simulink model "DDCU_wxt_v02_forA_OpenLoop"  (R2014a)
settings: Solver=FixedStepDiscrete  StartTime=0.0  StopTime=16  FixedStep=0.05  RelTol=1e-3
InitFcn:
  | Veh_Par_wxt
values from neighbouring files (symbols this model uses):
  ag_thr = 0.4*g    (= 3.924)    [Veh_Par_wxt.m]
  B = 2.25    [Veh_Par_wxt.m]
  bra_pre_em = 12    [Veh_Par_wxt.m]
  bra_pre_gz2 = 12/3    (= 4)    [Veh_Par_wxt.m]
  bra_pre_gz34 = 12/3    (= 4)    [Veh_Par_wxt.m]
  bra_pre_yd = 12/2    (= 6)    [Veh_Par_wxt.m]
  brakepre_dem_data = [0 1 2 3 4 5 6 7 8 9 10 11 12]    [Veh_Par_wxt.m]
  brakeTrq_dem_data = [0 218.198 436.396 654.594 872.792 1090.99 1309.188 1527.386 1745.584 1963.782 2181.98 2400.178 2618.376]    [Veh_Par_wxt.m]
  bratrq_max = 4*2618.376    (= 10473.504)    [Veh_Par_wxt.m]
  eff_tran = 0.75    [Veh_Par_wxt.m]
  G = Mass*g    (= 36297)    [Veh_Par_wxt.m]
  kd1 = 1    [Veh_Par_wxt.m]
  kd2 = 1    [Veh_Par_wxt.m]
  kd3 = 1    [Veh_Par_wxt.m]
  ki1 = 1    [Veh_Par_wxt.m]
  ki2 = 1    [Veh_Par_wxt.m]
  ki3 = 1    [Veh_Par_wxt.m]
  kp1 = 1    [Veh_Par_wxt.m]
  kp2 = 1    [Veh_Par_wxt.m]
  kp3 = 1    [Veh_Par_wxt.m]
  L = 3.12    [Veh_Par_wxt.m]
  premax = 12    [Veh_Par_wxt.m]
  Radius = 0.20    (= 0.2)    [Veh_Par_wxt.m]
  s_opt_yi_add = 0.05    [Veh_Par_wxt.m]
  s_opt_zhuan_add = 0.05    [Veh_Par_wxt.m]
  spd_map_mot = [0 100 200 300 360 400 500 600 700 800 900]*tras_ratio    [Veh_Par_wxt.m]
  spdmax = 900*tras_ratio    (= 5580)    [Veh_Par_wxt.m]
  speed_thr_park = 5/3.6/Radius*30/pi    (= 66.3145596216)    [Veh_Par_wxt.m]
  tras_ratio = 6.2    [Veh_Par_wxt.m]
  trq_map_mot = [1200 1200 1200 1200 1200 1080 864 720 617 540 480]/tras_ratio    [Veh_Par_wxt.m]
  trqmax = 80    [Veh_Par_wxt.m]
  v_thr1_b = 5    [Veh_Par_wxt.m]
  v_thr2_b = 20    [Veh_Par_wxt.m]
  v_thr_park = 5    [Veh_Par_wxt.m]
undefined symbols (not defined in the file or in its folder): DiscIntNeverNeededParam, sigbuilder_block
libraries: simulink x169, ec5744lib x9
(part 11 of 13)

== system DDCU_wxt_v02_forA_OpenLoop/MainControl/mode_control/backward/backward/Drive/驱动防滑控制TCS/转向TCS/右转/无滑转 ==
  trq_dem_lf : Inport
  trq_dem_lr : Inport  Port=2
  trq_dem_rf : Inport  Port=3
  trq_dem_rr : Inport  Port=4
  bra_pre_l : Inport  Port=5
  bra_pre_r : Inport  Port=6
  brake_dem : Inport  Port=7
  Action Port : ActionPort  ActionType=case
  1-D Lookup Table : Lookup_n-D  NumberOfTableDimensions=1  BreakpointsForDimension1=brakeTrq_dem_data  Table=brakepre_dem_data  InternalRulePriority=Speed  RndMeth=Simplest  InputSameDT=on
  1-D Lookup Table2 : Lookup_n-D  NumberOfTableDimensions=1  BreakpointsForDimension1=brakeTrq_dem_data  Table=brakepre_dem_data  InternalRulePriority=Speed  RndMeth=Simplest  InputSameDT=on
  Add2 : Sum
  Add3 : Sum
  Constant : Constant  Value=bratrq_max
  Gain1 : Gain  Gain=1/2
  Gain2 : Gain  Gain=1/100
  Gain3 : Gain  Gain=1/2
  Gain4 : Gain  Gain=1/2
  HeartBeat : MATLAB Function  TreatAsAtomicUnit=on
  HeartBeat1 : MATLAB Function  TreatAsAtomicUnit=on
  Memory : Memory  InheritSampleTime=on
  Memory1 : Memory  InheritSampleTime=on
  Mux : Mux  Inputs=8
  Mux1 : Mux  Inputs=8
  Mux2 : Mux  Inputs=7
  Mux3 : Mux  Inputs=7
  Product : Product
  Saturation{,1..3} (4 alike) : Saturate  UpperLimit=trqmax  LowerLimit=-trqmax
  Saturation4 : Saturate  UpperLimit=premax  LowerLimit=0
  Saturation5 : Saturate  UpperLimit=premax  LowerLimit=0
  SpdLim_dem{,1..3} (4 alike) : Constant  Value=spdmax
  SpdSet_dem{,1..3} (4 alike) : Constant
  TrqLim_dem{,1..3} (4 alike) : Constant
  mot_drive : Constant  Value=2
  mot_drive1 : Constant
  mot_drive2 : Constant  Value=2
  mot_drive3 : Constant
  mot_enable{,1..3} (4 alike) : Constant  Value=2
  mot_mode{,1..3} (4 alike) : Constant
  mot_lf : Outport
  mot_lr : Outport  Port=2
  mot_rf : Outport  Port=3
  mot_rr : Outport  Port=4
  bra_pre_l1 : Outport  Port=5
  bra_pre_r1 : Outport  Port=6
  wires:
  Saturation5/1 -> bra_pre_r1/1
  Saturation4/1 -> bra_pre_l1/1
  Saturation3/1 -> Mux3/4
  Saturation2/1 -> Mux2/4
  Saturation1/1 -> Mux1/4
  Saturation/1 -> Mux/4
  brake_dem/1 -> Gain2/1
  Add3/1 -> Saturation5/1
  bra_pre_r/1 -> Add3/2
  1-D Lookup Table2/1 -> Add3/1
  Gain4/1 -> 1-D Lookup Table2/1
  Gain3/1 -> 1-D Lookup Table/1
  Gain2/1 -> Product/2
  Gain1/1 -> Gain3/1, Gain4/1
  Product/1 -> Gain1/1
  Constant/1 -> Product/1
  1-D Lookup Table/1 -> Add2/1
  Add2/1 -> Saturation4/1
  bra_pre_l/1 -> Add2/2
  mot_drive/1 -> Mux/3
  mot_mode/1 -> Mux/2
  trq_dem_lf/1 -> Saturation/1
  mot_enable/1 -> Mux/1
  SpdSet_dem/1 -> Mux/5
  Mux/1 -> mot_lf/1
  TrqLim_dem/1 -> Mux/6
  HeartBeat/1(life) -> Mux/8, Memory/1
  Memory/1 -> HeartBeat/1(life_pre)
  SpdLim_dem/1 -> Mux/7
  mot_drive1/1 -> Mux2/3
  mot_mode2/1 -> Mux2/2
  trq_dem_rf/1 -> Saturation2/1
  mot_enable2/1 -> Mux2/1
  SpdSet_dem1/1 -> Mux2/5
  Mux2/1 -> mot_rf/1
  TrqLim_dem1/1 -> Mux2/6
  SpdLim_dem1/1 -> Mux2/7
  mot_drive2/1 -> Mux1/3
  mot_mode1/1 -> Mux1/2
  trq_dem_lr/1 -> Saturation1/1
  mot_enable1/1 -> Mux1/1
  SpdSet_dem2/1 -> Mux1/5
  Mux1/1 -> mot_lr/1
  TrqLim_dem2/1 -> Mux1/6
  HeartBeat1/1(life) -> Mux1/8, Memory1/1
  Memory1/1 -> HeartBeat1/1(life_pre)
  SpdLim_dem2/1 -> Mux1/7
  mot_drive3/1 -> Mux3/3
  mot_mode3/1 -> Mux3/2
  trq_dem_rr/1 -> Saturation3/1
  mot_enable3/1 -> Mux3/1
  SpdSet_dem3/1 -> Mux3/5
  Mux3/1 -> mot_rr/1
  TrqLim_dem3/1 -> Mux3/6
  SpdLim_dem3/1 -> Mux3/7

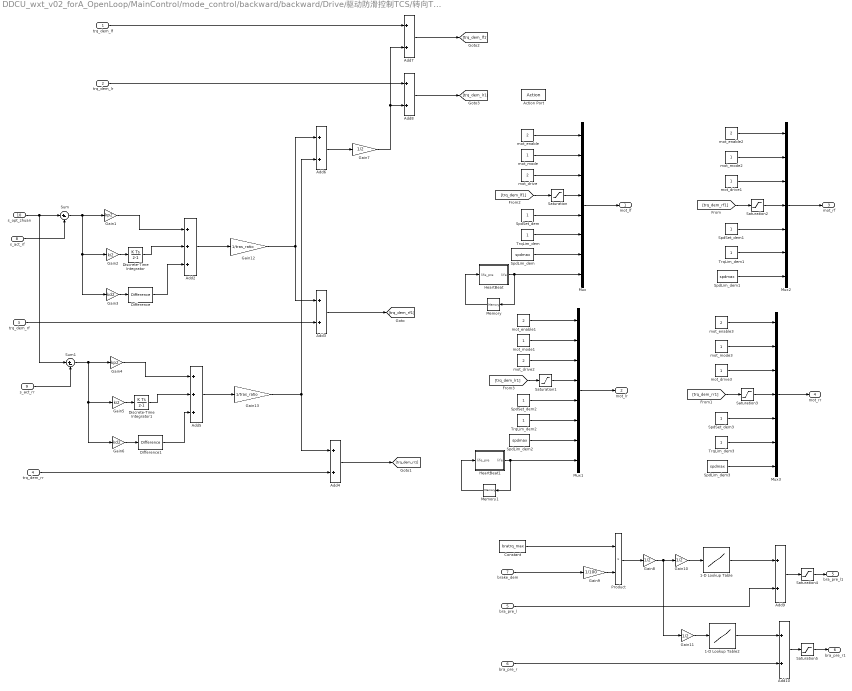
== system DDCU_wxt_v02_forA_OpenLoop/MainControl/mode_control/backward/backward/Drive/驱动防滑控制TCS/转向TCS/左转/前后轮均滑转 ==
  trq_dem_lf : Inport
  trq_dem_lr : Inport  Port=2
  trq_dem_rf : Inport  Port=3
  trq_dem_rr : Inport  Port=4
  bra_pre_l : Inport  Port=5
  bra_pre_r : Inport  Port=6
  brake_dem : Inport  Port=7
  s_act_rf : Inport  Port=8
  s_act_rr : Inport  Port=9
  s_opt_zhuan : Inport  Port=10
  Action Port : ActionPort  ActionType=case
  1-D Lookup Table : Lookup_n-D  NumberOfTableDimensions=1  BreakpointsForDimension1=brakeTrq_dem_data  Table=brakepre_dem_data  InternalRulePriority=Speed  RndMeth=Simplest  InputSameDT=on
  1-D Lookup Table2 : Lookup_n-D  NumberOfTableDimensions=1  BreakpointsForDimension1=brakeTrq_dem_data  Table=brakepre_dem_data  InternalRulePriority=Speed  RndMeth=Simplest  InputSameDT=on
  Add{3..4,6..10} (7 alike) : Sum
  Add2 : Sum  Inputs=+++
  Add5 : Sum  Inputs=+++
  Constant : Constant  Value=bratrq_max
  Difference : simulink/Discrete/Difference  ICPrevInput=0.0  InputProcessing=Inherited  OutMin=[]  OutMax=[]  OutDataType=fixdt(1, 16)  OutScaling=2^-10  DoSatur=off
  Difference1 : simulink/Discrete/Difference  ICPrevInput=0.0  InputProcessing=Inherited  OutMin=[]  OutMax=[]  OutDataType=fixdt(1, 16)  OutScaling=2^-10  DoSatur=off
  Discrete-Time Integrator : DiscreteIntegrator  SampleTime=-1  ICPrevOutput=DiscIntNeverNeededParam  ICPrevScaledInput=DiscIntNeverNeededParam
  Discrete-Time Integrator1 : DiscreteIntegrator  SampleTime=-1  ICPrevOutput=DiscIntNeverNeededParam  ICPrevScaledInput=DiscIntNeverNeededParam
  Gain1 : Gain  Gain=kp2
  Gain{7..8,10..11} (4 alike) : Gain  Gain=1/2
  Gain12 : Gain  Gain=1/tras_ratio
  Gain13 : Gain  Gain=1/tras_ratio
  Gain2 : Gain  Gain=ki2
  Gain3 : Gain  Gain=kd2
  Gain4 : Gain  Gain=kp2
  Gain5 : Gain  Gain=ki2
  Gain6 : Gain  Gain=kd2
  Gain9 : Gain  Gain=1/100
  HeartBeat : MATLAB Function  TreatAsAtomicUnit=on
  HeartBeat1 : MATLAB Function  TreatAsAtomicUnit=on
  Memory : Memory  InheritSampleTime=on
  Memory1 : Memory  InheritSampleTime=on
  Mux : Mux  Inputs=8
  Mux1 : Mux  Inputs=8
  Mux2 : Mux  Inputs=7
  Mux3 : Mux  Inputs=7
  Product : Product
  Saturation{,1..3} (4 alike) : Saturate  UpperLimit=trqmax  LowerLimit=-trqmax
  Saturation4 : Saturate  UpperLimit=premax  LowerLimit=0
  Saturation5 : Saturate  UpperLimit=premax  LowerLimit=0
  SpdLim_dem{,1..3} (4 alike) : Constant  Value=spdmax
  SpdSet_dem{,1..3} (4 alike) : Constant
  Sum : Sum  Inputs=|+-
  Sum1 : Sum  Inputs=|+-
  TrqLim_dem{,1..3} (4 alike) : Constant
  mot_drive : Constant  Value=2
  mot_drive1 : Constant
  mot_drive2 : Constant  Value=2
  mot_drive3 : Constant
  mot_enable{,1..3} (4 alike) : Constant  Value=2
  mot_mode{,1..3} (4 alike) : Constant
  mot_lf : Outport
  mot_lr : Outport  Port=2
  mot_rf : Outport  Port=3
  mot_rr : Outport  Port=4
  bra_pre_l1 : Outport  Port=5
  bra_pre_r1 : Outport  Port=6
  wires:
  Saturation5/1 -> bra_pre_r1/1
  Saturation4/1 -> bra_pre_l1/1
  Saturation3/1 -> Mux3/4
  Saturation2/1 -> Mux2/4
  Saturation1/1 -> Mux1/4
  Saturation/1 -> Mux/4
  Difference1/1 -> Add5/3
  Discrete-Time Integrator1/1 -> Add5/2
  Difference/1 -> Add2/3
  Discrete-Time Integrator/1 -> Add2/2
  brake_dem/1 -> Gain9/1
  Add10/1 -> Saturation5/1
  bra_pre_r/1 -> Add10/2
  1-D Lookup Table2/1 -> Add10/1
  Gain11/1 -> 1-D Lookup Table2/1
  Gain10/1 -> 1-D Lookup Table/1
  Gain9/1 -> Product/2
  Gain8/1 -> Gain10/1, Gain11/1
  Product/1 -> Gain8/1
  Constant/1 -> Product/1
  1-D Lookup Table/1 -> Add9/1
  Add9/1 -> Saturation4/1
  bra_pre_l/1 -> Add9/2
  Add8/1 -> [trq_dem_lr1]
  trq_dem_lr/1 -> Add8/1
  Add7/1 -> [trq_dem_lf1]
  Gain7/1 -> Add7/2, Add8/2
  trq_dem_lf/1 -> Add7/1
  Add6/1 -> Gain7/1
  trq_dem_rr/1 -> Add4/2
  Add5/1 -> Gain13/1
  s_act_rr/1 -> Sum1/2
  Gain6/1 -> Difference1/1
  Gain5/1 -> Discrete-Time Integrator1/1
  Gain4/1 -> Add5/1
  Sum1/1 -> Gain4/1, Gain6/1, Gain5/1
  Add4/1 -> [trq_dem_rr1]
  Add3/1 -> [trq_dem_rf1]
  trq_dem_rf/1 -> Add3/2
  Add2/1 -> Gain12/1
  s_act_rf/1 -> Sum/2
  Gain3/1 -> Difference/1
  Gain2/1 -> Discrete-Time Integrator/1
  Gain1/1 -> Add2/1
  Sum/1 -> Gain1/1, Gain3/1, Gain2/1
  s_opt_zhuan/1 -> Sum/1, Sum1/1
  mot_drive/1 -> Mux/3
  mot_mode/1 -> Mux/2
  [trq_dem_lf1] -> Saturation/1
  mot_enable/1 -> Mux/1
  SpdSet_dem/1 -> Mux/5
  Mux/1 -> mot_lf/1
  TrqLim_dem/1 -> Mux/6
  HeartBeat/1(life) -> Mux/8, Memory/1
  Memory/1 -> HeartBeat/1(life_pre)
  SpdLim_dem/1 -> Mux/7
  mot_drive1/1 -> Mux2/3
  mot_mode2/1 -> Mux2/2
  [trq_dem_rf1] -> Saturation2/1
  mot_enable2/1 -> Mux2/1
  SpdSet_dem1/1 -> Mux2/5
  Mux2/1 -> mot_rf/1
  TrqLim_dem1/1 -> Mux2/6
  SpdLim_dem1/1 -> Mux2/7
  mot_drive2/1 -> Mux1/3
  mot_mode1/1 -> Mux1/2
  [trq_dem_lr1] -> Saturation1/1
  mot_enable1/1 -> Mux1/1
  SpdSet_dem2/1 -> Mux1/5
  Mux1/1 -> mot_lr/1
  TrqLim_dem2/1 -> Mux1/6
  HeartBeat1/1(life) -> Mux1/8, Memory1/1
  Memory1/1 -> HeartBeat1/1(life_pre)
  SpdLim_dem2/1 -> Mux1/7
  mot_drive3/1 -> Mux3/3
  mot_mode3/1 -> Mux3/2
  [trq_dem_rr1] -> Saturation3/1
  mot_enable3/1 -> Mux3/1
  SpdSet_dem3/1 -> Mux3/5
  Mux3/1 -> mot_rr/1
  TrqLim_dem3/1 -> Mux3/6
  SpdLim_dem3/1 -> Mux3/7
  Gain12/1 -> Add6/1, Add3/1
  Gain13/1 -> Add6/2, Add4/1

== system DDCU_wxt_v02_forA_OpenLoop/MainControl/mode_control/backward/backward/Drive/驱动防滑控制TCS/转向TCS/左转/前轮滑转 ==
  trq_dem_lf : Inport
  trq_dem_lr : Inport  Port=2
  trq_dem_rf : Inport  Port=3
  trq_dem_rr : Inport  Port=4
  bra_pre_l : Inport  Port=5
  bra_pre_r : Inport  Port=6
  brake_dem : Inport  Port=7
  s_act_rf : Inport  Port=8
  s_opt_zhuan : Inport  Port=9
  Action Port : ActionPort  ActionType=case
  1-D Lookup Table : Lookup_n-D  NumberOfTableDimensions=1  BreakpointsForDimension1=brakeTrq_dem_data  Table=brakepre_dem_data  InternalRulePriority=Speed  RndMeth=Simplest  InputSameDT=on
  1-D Lookup Table2 : Lookup_n-D  NumberOfTableDimensions=1  BreakpointsForDimension1=brakeTrq_dem_data  Table=brakepre_dem_data  InternalRulePriority=Speed  RndMeth=Simplest  InputSameDT=on
  Add2 : Sum  Inputs=+++
  Add{3..6} (4 alike) : Sum
  Constant : Constant  Value=bratrq_max
  Difference : simulink/Discrete/Difference  ICPrevInput=0.0  InputProcessing=Inherited  OutMin=[]  OutMax=[]  OutDataType=fixdt(1, 16)  OutScaling=2^-10  DoSatur=off
  Discrete-Time Integrator : DiscreteIntegrator  SampleTime=-1  ICPrevOutput=DiscIntNeverNeededParam  ICPrevScaledInput=DiscIntNeverNeededParam
  Gain1 : Gain  Gain=kp2
  Gain2 : Gain  Gain=ki2
  Gain3 : Gain  Gain=kd2
  Gain4 : Gain  Gain=-1
  Gain5 : Gain  Gain=1/2
  Gain6 : Gain  Gain=1/100
  Gain7 : Gain  Gain=1/2
  Gain8 : Gain  Gain=1/2
  Gain9 : Gain  Gain=1/tras_ratio
  HeartBeat : MATLAB Function  TreatAsAtomicUnit=on
  HeartBeat1 : MATLAB Function  TreatAsAtomicUnit=on
  Memory : Memory  InheritSampleTime=on
  Memory1 : Memory  InheritSampleTime=on
  Mux : Mux  Inputs=8
  Mux1 : Mux  Inputs=8
  Mux2 : Mux  Inputs=7
  Mux3 : Mux  Inputs=7
  Product : Product
  Saturation{,1..3} (4 alike) : Saturate  UpperLimit=trqmax  LowerLimit=-trqmax
  Saturation4 : Saturate  UpperLimit=premax  LowerLimit=0
  Saturation5 : Saturate  UpperLimit=premax  LowerLimit=0
  SpdLim_dem{,1..3} (4 alike) : Constant  Value=spdmax
  SpdSet_dem{,1..3} (4 alike) : Constant
  Sum : Sum  Inputs=|+-
  TrqLim_dem{,1..3} (4 alike) : Constant
  mot_drive : Constant  Value=2
  mot_drive1 : Constant
  mot_drive2 : Constant  Value=2
  mot_drive3 : Constant
  mot_enable{,1..3} (4 alike) : Constant  Value=2
  mot_mode{,1..3} (4 alike) : Constant
  mot_lf : Outport
  mot_lr : Outport  Port=2
  mot_rf : Outport  Port=3
  mot_rr : Outport  Port=4
  bra_pre_l1 : Outport  Port=5
  bra_pre_r1 : Outport  Port=6
  wires:
  Saturation5/1 -> bra_pre_r1/1
  Saturation4/1 -> bra_pre_l1/1
  Saturation3/1 -> Mux3/4
  Saturation2/1 -> Mux2/4
  Saturation1/1 -> Mux1/4
  Saturation/1 -> Mux/4
  Difference/1 -> Add2/3
  Discrete-Time Integrator/1 -> Add2/2
  brake_dem/1 -> Gain6/1
  Add6/1 -> Saturation5/1
  bra_pre_r/1 -> Add6/2
  1-D Lookup Table2/1 -> Add6/1
  Gain8/1 -> 1-D Lookup Table2/1
  Gain7/1 -> 1-D Lookup Table/1
  Gain6/1 -> Product/2
  Gain5/1 -> Gain7/1, Gain8/1
  Product/1 -> Gain5/1
  Constant/1 -> Product/1
  1-D Lookup Table/1 -> Add5/1
  Add5/1 -> Saturation4/1
  bra_pre_l/1 -> Add5/2
  Add4/1 -> [trq_dem_rr1]
  trq_dem_rr/1 -> Add4/2
  Gain4/1 -> Add4/1
  Add3/1 -> [trq_dem_rf1]
  trq_dem_rf/1 -> Add3/2
  Add2/1 -> Gain9/1
  s_act_rf/1 -> Sum/2
  Gain3/1 -> Difference/1
  Gain2/1 -> Discrete-Time Integrator/1
  Gain1/1 -> Add2/1
  Sum/1 -> Gain1/1, Gain3/1, Gain2/1
  s_opt_zhuan/1 -> Sum/1
  mot_drive/1 -> Mux/3
  mot_mode/1 -> Mux/2
  trq_dem_lf/1 -> Saturation/1
  mot_enable/1 -> Mux/1
  SpdSet_dem/1 -> Mux/5
  Mux/1 -> mot_lf/1
  TrqLim_dem/1 -> Mux/6
  HeartBeat/1(life) -> Mux/8, Memory/1
  Memory/1 -> HeartBeat/1(life_pre)
  SpdLim_dem/1 -> Mux/7
  mot_drive1/1 -> Mux2/3
  mot_mode2/1 -> Mux2/2
  [trq_dem_rf1] -> Saturation2/1
  mot_enable2/1 -> Mux2/1
  SpdSet_dem1/1 -> Mux2/5
  Mux2/1 -> mot_rf/1
  TrqLim_dem1/1 -> Mux2/6
  SpdLim_dem1/1 -> Mux2/7
  mot_drive2/1 -> Mux1/3
  mot_mode1/1 -> Mux1/2
  trq_dem_lr/1 -> Saturation1/1
  mot_enable1/1 -> Mux1/1
  SpdSet_dem2/1 -> Mux1/5
  Mux1/1 -> mot_lr/1
  TrqLim_dem2/1 -> Mux1/6
  HeartBeat1/1(life) -> Mux1/8, Memory1/1
  Memory1/1 -> HeartBeat1/1(life_pre)
  SpdLim_dem2/1 -> Mux1/7
  mot_drive3/1 -> Mux3/3
  mot_mode3/1 -> Mux3/2
  [trq_dem_rr1] -> Saturation3/1
  mot_enable3/1 -> Mux3/1
  SpdSet_dem3/1 -> Mux3/5
  Mux3/1 -> mot_rr/1
  TrqLim_dem3/1 -> Mux3/6
  SpdLim_dem3/1 -> Mux3/7
  Gain9/1 -> Add3/1, Gain4/1

== system DDCU_wxt_v02_forA_OpenLoop/MainControl/mode_control/backward/backward/Drive/驱动防滑控制TCS/转向TCS/左转/后轮滑转 ==
  trq_dem_lf : Inport
  trq_dem_lr : Inport  Port=2
  trq_dem_rf : Inport  Port=3
  trq_dem_rr : Inport  Port=4
  bra_pre_l : Inport  Port=5
  bra_pre_r : Inport  Port=6
  brake_dem : Inport  Port=7
  s_act_rr : Inport  Port=8
  s_opt_zhuan : Inport  Port=9
  Action Port : ActionPort  ActionType=case
  1-D Lookup Table : Lookup_n-D  NumberOfTableDimensions=1  BreakpointsForDimension1=brakeTrq_dem_data  Table=brakepre_dem_data  InternalRulePriority=Speed  RndMeth=Simplest  InputSameDT=on
  1-D Lookup Table2 : Lookup_n-D  NumberOfTableDimensions=1  BreakpointsForDimension1=brakeTrq_dem_data  Table=brakepre_dem_data  InternalRulePriority=Speed  RndMeth=Simplest  InputSameDT=on
  Add2 : Sum  Inputs=+++
  Add{3..6} (4 alike) : Sum
  Constant : Constant  Value=bratrq_max
  Difference : simulink/Discrete/Difference  ICPrevInput=0.0  InputProcessing=Inherited  OutMin=[]  OutMax=[]  OutDataType=fixdt(1, 16)  OutScaling=2^-10  DoSatur=off
  Discrete-Time Integrator : DiscreteIntegrator  SampleTime=-1  ICPrevOutput=DiscIntNeverNeededParam  ICPrevScaledInput=DiscIntNeverNeededParam
  Gain1 : Gain  Gain=kp2
  Gain2 : Gain  Gain=ki2
  Gain3 : Gain  Gain=kd2
  Gain4 : Gain  Gain=-1
  Gain5 : Gain  Gain=1/2
  Gain6 : Gain  Gain=1/100
  Gain7 : Gain  Gain=1/2
  Gain8 : Gain  Gain=1/2
  Gain9 : Gain  Gain=1/tras_ratio
  HeartBeat : MATLAB Function  TreatAsAtomicUnit=on
  HeartBeat1 : MATLAB Function  TreatAsAtomicUnit=on
  Memory : Memory  InheritSampleTime=on
  Memory1 : Memory  InheritSampleTime=on
  Mux : Mux  Inputs=8
  Mux1 : Mux  Inputs=8
  Mux2 : Mux  Inputs=7
  Mux3 : Mux  Inputs=7
  Product : Product
  Saturation{,1..3} (4 alike) : Saturate  UpperLimit=trqmax  LowerLimit=-trqmax
  Saturation4 : Saturate  UpperLimit=premax  LowerLimit=0
  Saturation5 : Saturate  UpperLimit=premax  LowerLimit=0
  SpdLim_dem{,1..3} (4 alike) : Constant  Value=spdmax
  SpdSet_dem{,1..3} (4 alike) : Constant
  Sum : Sum  Inputs=|+-
  TrqLim_dem{,1..3} (4 alike) : Constant
  mot_drive : Constant  Value=2
  mot_drive1 : Constant
  mot_drive2 : Constant  Value=2
  mot_drive3 : Constant
  mot_enable{,1..3} (4 alike) : Constant  Value=2
  mot_mode{,1..3} (4 alike) : Constant
  mot_lf : Outport
  mot_lr : Outport  Port=2
  mot_rf : Outport  Port=3
  mot_rr : Outport  Port=4
  bra_pre_l1 : Outport  Port=5
  bra_pre_r1 : Outport  Port=6
  wires:
  Saturation5/1 -> bra_pre_r1/1
  Saturation4/1 -> bra_pre_l1/1
  Saturation3/1 -> Mux3/4
  Saturation2/1 -> Mux1/4
  Saturation1/1 -> Mux2/4
  Saturation/1 -> Mux/4
  Difference/1 -> Add2/3
  Discrete-Time Integrator/1 -> Add2/2
  brake_dem/1 -> Gain6/1
  Add6/1 -> Saturation5/1
  bra_pre_r/1 -> Add6/2
  1-D Lookup Table2/1 -> Add6/1
  Gain8/1 -> 1-D Lookup Table2/1
  Gain7/1 -> 1-D Lookup Table/1
  Gain6/1 -> Product/2
  Gain5/1 -> Gain7/1, Gain8/1
  Product/1 -> Gain5/1
  Constant/1 -> Product/1
  1-D Lookup Table/1 -> Add5/1
  Add5/1 -> Saturation4/1
  bra_pre_l/1 -> Add5/2
  SpdLim_dem3/1 -> Mux3/7
  TrqLim_dem3/1 -> Mux3/6
  Mux3/1 -> mot_rr/1
  SpdSet_dem3/1 -> Mux3/5
  mot_enable3/1 -> Mux3/1
  [trq_dem_rr1] -> Saturation3/1
  mot_mode3/1 -> Mux3/2
  mot_drive3/1 -> Mux3/3
  SpdLim_dem2/1 -> Mux1/7
  Memory1/1 -> HeartBeat1/1(life_pre)
  HeartBeat1/1(life) -> Memory1/1, Mux1/8
  TrqLim_dem2/1 -> Mux1/6
  Mux1/1 -> mot_lr/1
  SpdSet_dem2/1 -> Mux1/5
  mot_enable1/1 -> Mux1/1
  trq_dem_lr/1 -> Saturation2/1
  mot_mode1/1 -> Mux1/2
  mot_drive2/1 -> Mux1/3
  SpdLim_dem1/1 -> Mux2/7
  TrqLim_dem1/1 -> Mux2/6
  Mux2/1 -> mot_rf/1
  SpdSet_dem1/1 -> Mux2/5
  mot_enable2/1 -> Mux2/1
  [trq_dem_rf1] -> Saturation1/1
  mot_mode2/1 -> Mux2/2
  mot_drive1/1 -> Mux2/3
  SpdLim_dem/1 -> Mux/7
  Memory/1 -> HeartBeat/1(life_pre)
  HeartBeat/1(life) -> Memory/1, Mux/8
  TrqLim_dem/1 -> Mux/6
  Mux/1 -> mot_lf/1
  SpdSet_dem/1 -> Mux/5
  mot_enable/1 -> Mux/1
  trq_dem_lf/1 -> Saturation/1
  mot_mode/1 -> Mux/2
  mot_drive/1 -> Mux/3
  s_opt_zhuan/1 -> Sum/1
  Sum/1 -> Gain2/1, Gain3/1, Gain1/1
  Gain1/1 -> Add2/1
  Gain2/1 -> Discrete-Time Integrator/1
  Gain3/1 -> Difference/1
  s_act_rr/1 -> Sum/2
  Add2/1 -> Gain9/1
  trq_dem_rr/1 -> Add3/2
  Add3/1 -> [trq_dem_rr1]
  Gain4/1 -> Add4/1
  trq_dem_rf/1 -> Add4/2
  Add4/1 -> [trq_dem_rf1]
  Gain9/1 -> Gain4/1, Add3/1

== system DDCU_wxt_v02_forA_OpenLoop/MainControl/mode_control/backward/backward/Drive/驱动防滑控制TCS/转向TCS/左转/无滑转 ==
  trq_dem_lf : Inport
  trq_dem_lr : Inport  Port=2
  trq_dem_rf : Inport  Port=3
  trq_dem_rr : Inport  Port=4
  bra_pre_l : Inport  Port=5
  bra_pre_r : Inport  Port=6
  brake_dem : Inport  Port=7
  Action Port : ActionPort  ActionType=case
  1-D Lookup Table : Lookup_n-D  NumberOfTableDimensions=1  BreakpointsForDimension1=brakeTrq_dem_data  Table=brakepre_dem_data  InternalRulePriority=Speed  RndMeth=Simplest  InputSameDT=on
  1-D Lookup Table2 : Lookup_n-D  NumberOfTableDimensions=1  BreakpointsForDimension1=brakeTrq_dem_data  Table=brakepre_dem_data  InternalRulePriority=Speed  RndMeth=Simplest  InputSameDT=on
  Add : Sum
  Add2 : Sum
  Constant : Constant  Value=bratrq_max
  Gain1 : Gain  Gain=1/2
  Gain2 : Gain  Gain=1/100
  Gain3 : Gain  Gain=1/2
  Gain4 : Gain  Gain=1/2
  HeartBeat : MATLAB Function  TreatAsAtomicUnit=on
  HeartBeat1 : MATLAB Function  TreatAsAtomicUnit=on
  Memory : Memory  InheritSampleTime=on
  Memory1 : Memory  InheritSampleTime=on
  Mux : Mux  Inputs=8
  Mux1 : Mux  Inputs=8
  Mux2 : Mux  Inputs=7
  Mux3 : Mux  Inputs=7
  Product : Product
  Saturation{,1..3} (4 alike) : Saturate  UpperLimit=trqmax  LowerLimit=-trqmax
  Saturation4 : Saturate  UpperLimit=premax  LowerLimit=0
  Saturation5 : Saturate  UpperLimit=premax  LowerLimit=0
  SpdLim_dem{,1..3} (4 alike) : Constant  Value=spdmax
  SpdSet_dem{,1..3} (4 alike) : Constant
  TrqLim_dem{,1..3} (4 alike) : Constant
  mot_drive : Constant  Value=2
  mot_drive1 : Constant
  mot_drive2 : Constant  Value=2
  mot_drive3 : Constant
  mot_enable{,1..3} (4 alike) : Constant  Value=2
  mot_mode{,1..3} (4 alike) : Constant
  mot_lf : Outport
  mot_lr : Outport  Port=2
  mot_rf : Outport  Port=3
  mot_rr : Outport  Port=4
  bra_pre_l1 : Outport  Port=5
  bra_pre_r1 : Outport  Port=6
  wires:
  Saturation5/1 -> bra_pre_r1/1
  Saturation4/1 -> bra_pre_l1/1
  Saturation3/1 -> Mux3/4
  Saturation2/1 -> Mux2/4
  Saturation1/1 -> Mux1/4
  Saturation/1 -> Mux/4
  brake_dem/1 -> Gain2/1
  Add2/1 -> Saturation5/1
  bra_pre_r/1 -> Add2/2
  1-D Lookup Table2/1 -> Add2/1
  Gain4/1 -> 1-D Lookup Table2/1
  Gain3/1 -> 1-D Lookup Table/1
  Gain2/1 -> Product/2
  Gain1/1 -> Gain3/1, Gain4/1
  Product/1 -> Gain1/1
  Constant/1 -> Product/1
  1-D Lookup Table/1 -> Add/1
  Add/1 -> Saturation4/1
  bra_pre_l/1 -> Add/2
  SpdLim_dem3/1 -> Mux3/7
  TrqLim_dem3/1 -> Mux3/6
  Mux3/1 -> mot_rr/1
  SpdSet_dem3/1 -> Mux3/5
  mot_enable3/1 -> Mux3/1
  trq_dem_rr/1 -> Saturation3/1
  mot_mode3/1 -> Mux3/2
  mot_drive3/1 -> Mux3/3
  SpdLim_dem2/1 -> Mux1/7
  Memory1/1 -> HeartBeat1/1(life_pre)
  HeartBeat1/1(life) -> Memory1/1, Mux1/8
  TrqLim_dem2/1 -> Mux1/6
  Mux1/1 -> mot_lr/1
  SpdSet_dem2/1 -> Mux1/5
  mot_enable1/1 -> Mux1/1
  trq_dem_lr/1 -> Saturation1/1
  mot_mode1/1 -> Mux1/2
  mot_drive2/1 -> Mux1/3
  SpdLim_dem1/1 -> Mux2/7
  TrqLim_dem1/1 -> Mux2/6
  Mux2/1 -> mot_rf/1
  SpdSet_dem1/1 -> Mux2/5
  mot_enable2/1 -> Mux2/1
  trq_dem_rf/1 -> Saturation2/1
  mot_mode2/1 -> Mux2/2
  mot_drive1/1 -> Mux2/3
  SpdLim_dem/1 -> Mux/7
  Memory/1 -> HeartBeat/1(life_pre)
  HeartBeat/1(life) -> Memory/1, Mux/8
  TrqLim_dem/1 -> Mux/6
  Mux/1 -> mot_lf/1
  SpdSet_dem/1 -> Mux/5
  mot_enable/1 -> Mux/1
  trq_dem_lf/1 -> Saturation/1
  mot_mode/1 -> Mux/2
  mot_drive/1 -> Mux/3

== system DDCU_wxt_v02_forA_OpenLoop/MainControl/mode_control/forward/forward/Drive/驱动防滑控制TCS/直行TCS/直行/Subsystem ==
  s_opt_zhuan : Inport
  s_act_lf : Inport  Port=2
  s_act_lr : Inport  Port=3
  s_act_rf : Inport  Port=4
  s_act_rr : Inport  Port=5
  flag_lf : Inport  Port=6
  flag_lr : Inport  Port=7
  flag_rf : Inport  Port=8
  flag_rr : Inport  Port=9
  trq_dem_lf : Inport  Port=10
  trq_dem_lr : Inport  Port=11
  trq_dem_rf : Inport  Port=12
  trq_dem_rr : Inport  Port=13
  Add{1..2,5,7} (4 alike) : Sum  Inputs=+++
  Add{3..4,6,8} (4 alike) : Sum
  Difference{,1..3} (4 alike) : simulink/Discrete/Difference  ICPrevInput=0.0  InputProcessing=Inherited  OutMin=[]  OutMax=[]  OutDataType=fixdt(1, 16)  OutScaling=2^-10  DoSatur=off
  Discrete-Time Integrator{,1..3} (4 alike) : DiscreteIntegrator  SampleTime=-1  ICPrevOutput=DiscIntNeverNeededParam  ICPrevScaledInput=DiscIntNeverNeededParam
  Gain{,13..15} (4 alike) : Gain  Gain=1/tras_ratio
  Gain{1,4,7,10} (4 alike) : Gain  Gain=kp2
  Gain{2,5,8,11} (4 alike) : Gain  Gain=ki2
  Gain{3,6,9,12} (4 alike) : Gain  Gain=kd2
  Sum{,1..3} (4 alike) : Sum  Inputs=|+-
  Switch{,1..3} (4 alike) : Switch  Criteria=u2 > Threshold  Threshold=0.5
  trq_pid_lf : Outport
  trq_pid_lr : Outport  Port=2
  trq_pid_rf : Outport  Port=3
  trq_pid_rr : Outport  Port=4
  wires:
  Add3/1 -> Switch/1
  trq_dem_lf/1 -> Switch/3, Add3/2
  s_act_lf/1 -> Sum/2
  Gain3/1 -> Difference/1
  Gain2/1 -> Discrete-Time Integrator/1
  Gain1/1 -> Add2/1
  s_opt_zhuan/1 -> [s_opt_zhuan], Sum/1
  flag_lf/1 -> Switch/2
  Switch/1 -> trq_pid_lf/1
  Add4/1 -> Switch1/1
  trq_dem_lr/1 -> Switch1/3, Add4/2
  s_act_lr/1 -> Sum1/2
  Gain5/1 -> Discrete-Time Integrator1/1
  Gain4/1 -> Add1/1
  [s_opt_zhuan] -> Sum1/1
  flag_lr/1 -> Switch1/2
  Switch1/1 -> trq_pid_lr/1
  Add6/1 -> Switch2/1
  trq_dem_rr/1 -> Switch2/3, Add6/2
  s_act_rr/1 -> Sum2/2
  Gain9/1 -> Difference2/1
  Gain8/1 -> Discrete-Time Integrator2/1
  Gain7/1 -> Add5/1
  [s_opt_zhuan] -> Sum2/1
  flag_rr/1 -> Switch2/2
  Switch2/1 -> trq_pid_rr/1
  Add8/1 -> Switch3/1
  trq_dem_rf/1 -> Switch3/3, Add8/2
  s_act_rf/1 -> Sum3/2
  Gain12/1 -> Difference3/1
  Gain11/1 -> Discrete-Time Integrator3/1
  Gain10/1 -> Add7/1
  [s_opt_zhuan] -> Sum3/1
  flag_rf/1 -> Switch3/2
  Switch3/1 -> trq_pid_rf/1
  Add2/1 -> Gain/1
  Sum/1 -> Gain2/1, Gain3/1, Gain1/1
  Sum1/1 -> Gain5/1, Gain6/1, Gain4/1
  Add1/1 -> Gain13/1
  Gain6/1 -> Difference1/1
  Add7/1 -> Gain14/1
  Sum3/1 -> Gain11/1, Gain12/1, Gain10/1
  Sum2/1 -> Gain8/1, Gain9/1, Gain7/1
  Add5/1 -> Gain15/1
  Discrete-Time Integrator/1 -> Add2/2
  Difference/1 -> Add2/3
  Discrete-Time Integrator1/1 -> Add1/2
  Difference1/1 -> Add1/3
  Discrete-Time Integrator3/1 -> Add7/2
  Difference3/1 -> Add7/3
  Discrete-Time Integrator2/1 -> Add5/2
  Difference2/1 -> Add5/3
  Gain/1 -> Add3/1
  Gain13/1 -> Add4/1
  Gain14/1 -> Add8/1
  Gain15/1 -> Add6/1

== system DDCU_wxt_v02_forA_OpenLoop/MainControl/mode_control/forward/forward/Drive/驱动防滑控制TCS/直行TCS/直行/Subsystem1 ==
  brake_dem : Inport
  1-D Lookup Table : Lookup_n-D  NumberOfTableDimensions=1  BreakpointsForDimension1=brakeTrq_dem_data  Table=brakepre_dem_data  InternalRulePriority=Speed  RndMeth=Simplest  InputSameDT=on
  Constant : Constant  Value=bratrq_max
  Gain1 : Gain  Gain=1/2
  Gain2 : Gain  Gain=1/100
  Gain3 : Gain  Gain=1/2
  Product : Product
  brakepre_dem : Outport
  wires:
  1-D Lookup Table/1 -> brakepre_dem/1
  Constant/1 -> Product/1
  Product/1 -> Gain1/1
  Gain1/1 -> Gain3/1
  Gain2/1 -> Product/2
  Gain3/1 -> 1-D Lookup Table/1
  brake_dem/1 -> Gain2/1

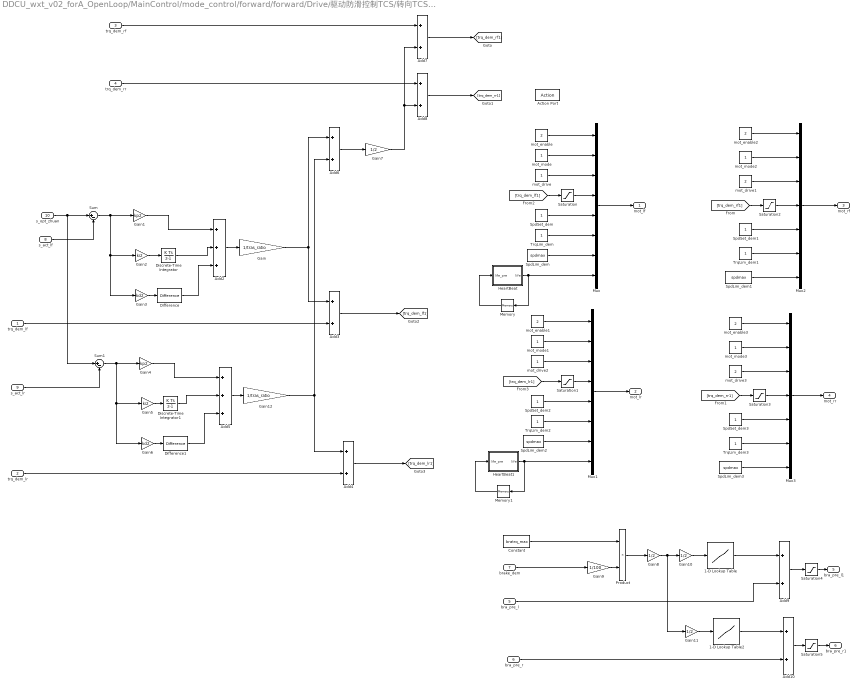
== system DDCU_wxt_v02_forA_OpenLoop/MainControl/mode_control/forward/forward/Drive/驱动防滑控制TCS/转向TCS/右转/前后轮均滑转 ==
  trq_dem_lf : Inport
  trq_dem_lr : Inport  Port=2
  trq_dem_rf : Inport  Port=3
  trq_dem_rr : Inport  Port=4
  bra_pre_l : Inport  Port=5
  bra_pre_r : Inport  Port=6
  brake_dem : Inport  Port=7
  s_act_lf : Inport  Port=8
  s_act_lr : Inport  Port=9
  s_opt_zhuan : Inport  Port=10
  Action Port : ActionPort  ActionType=case
  1-D Lookup Table : Lookup_n-D  NumberOfTableDimensions=1  BreakpointsForDimension1=brakeTrq_dem_data  Table=brakepre_dem_data  InternalRulePriority=Speed  RndMeth=Simplest  InputSameDT=on
  1-D Lookup Table2 : Lookup_n-D  NumberOfTableDimensions=1  BreakpointsForDimension1=brakeTrq_dem_data  Table=brakepre_dem_data  InternalRulePriority=Speed  RndMeth=Simplest  InputSameDT=on
  Add{3..4,6..10} (7 alike) : Sum
  Add2 : Sum  Inputs=+++
  Add5 : Sum  Inputs=+++
  Constant : Constant  Value=bratrq_max
  Difference : simulink/Discrete/Difference  ICPrevInput=0.0  InputProcessing=Inherited  OutMin=[]  OutMax=[]  OutDataType=fixdt(1, 16)  OutScaling=2^-10  DoSatur=off
  Difference1 : simulink/Discrete/Difference  ICPrevInput=0.0  InputProcessing=Inherited  OutMin=[]  OutMax=[]  OutDataType=fixdt(1, 16)  OutScaling=2^-10  DoSatur=off
  Discrete-Time Integrator : DiscreteIntegrator  SampleTime=-1  ICPrevOutput=DiscIntNeverNeededParam  ICPrevScaledInput=DiscIntNeverNeededParam
  Discrete-Time Integrator1 : DiscreteIntegrator  SampleTime=-1  ICPrevOutput=DiscIntNeverNeededParam  ICPrevScaledInput=DiscIntNeverNeededParam
  Gain : Gain  Gain=1/tras_ratio
  Gain1 : Gain  Gain=kp2
  Gain{7..8,10..11} (4 alike) : Gain  Gain=1/2
  Gain12 : Gain  Gain=1/tras_ratio
  Gain2 : Gain  Gain=ki2
  Gain3 : Gain  Gain=kd2
  Gain4 : Gain  Gain=kp2
  Gain5 : Gain  Gain=ki2
  Gain6 : Gain  Gain=kd2
  Gain9 : Gain  Gain=1/100
  HeartBeat : MATLAB Function  TreatAsAtomicUnit=on
  HeartBeat1 : MATLAB Function  TreatAsAtomicUnit=on
  Memory : Memory  InheritSampleTime=on
  Memory1 : Memory  InheritSampleTime=on
  Mux : Mux  Inputs=8
  Mux1 : Mux  Inputs=8
  Mux2 : Mux  Inputs=7
  Mux3 : Mux  Inputs=7
  Product : Product
  Saturation{,1..3} (4 alike) : Saturate  UpperLimit=trqmax  LowerLimit=-trqmax
  Saturation4 : Saturate  UpperLimit=premax  LowerLimit=0
  Saturation5 : Saturate  UpperLimit=premax  LowerLimit=0
  SpdLim_dem{,1..3} (4 alike) : Constant  Value=spdmax
  SpdSet_dem{,1..3} (4 alike) : Constant
  Sum : Sum  Inputs=|+-
  Sum1 : Sum  Inputs=|+-
  TrqLim_dem{,1..3} (4 alike) : Constant
  mot_drive : Constant
  mot_drive1 : Constant  Value=2
  mot_drive2 : Constant
  mot_drive3 : Constant  Value=2
  mot_enable{,1..3} (4 alike) : Constant  Value=2
  mot_mode{,1..3} (4 alike) : Constant
  mot_lf : Outport
  mot_lr : Outport  Port=2
  mot_rf : Outport  Port=3
  mot_rr : Outport  Port=4
  bra_pre_l1 : Outport  Port=5
  bra_pre_r1 : Outport  Port=6
  wires:
  Add8/1 -> [trq_dem_rr1]
  trq_dem_rr/1 -> Add8/1
  Add7/1 -> [trq_dem_rf1]
  Gain7/1 -> Add7/2, Add8/2
  trq_dem_rf/1 -> Add7/1
  Add6/1 -> Gain7/1
  trq_dem_lr/1 -> Add4/2
  Add5/1 -> Gain12/1
  s_act_lr/1 -> Sum1/2
  Gain6/1 -> Difference1/1
  Gain5/1 -> Discrete-Time Integrator1/1
  Gain4/1 -> Add5/1
  Sum1/1 -> Gain4/1, Gain6/1, Gain5/1
  Add4/1 -> [trq_dem_lr1]
  Add3/1 -> [trq_dem_lf1]
  trq_dem_lf/1 -> Add3/2
  Add2/1 -> Gain/1
  s_act_lf/1 -> Sum/2
  Gain2/1 -> Discrete-Time Integrator/1
  Gain1/1 -> Add2/1
  Sum/1 -> Gain1/1, Gain3/1, Gain2/1
  s_opt_zhuan/1 -> Sum/1, Sum1/1
  mot_drive/1 -> Mux/3
  mot_mode/1 -> Mux/2
  [trq_dem_lf1] -> Saturation/1
  mot_enable/1 -> Mux/1
  SpdSet_dem/1 -> Mux/5
  Mux/1 -> mot_lf/1
  TrqLim_dem/1 -> Mux/6
  HeartBeat/1(life) -> Mux/8, Memory/1
  Memory/1 -> HeartBeat/1(life_pre)
  SpdLim_dem/1 -> Mux/7
  mot_drive1/1 -> Mux2/3
  mot_mode2/1 -> Mux2/2
  [trq_dem_rf1] -> Saturation2/1
  mot_enable2/1 -> Mux2/1
  SpdSet_dem1/1 -> Mux2/5
  Mux2/1 -> mot_rf/1
  TrqLim_dem1/1 -> Mux2/6
  SpdLim_dem1/1 -> Mux2/7
  mot_drive2/1 -> Mux1/3
  mot_mode1/1 -> Mux1/2
  [trq_dem_lr1] -> Saturation1/1
  mot_enable1/1 -> Mux1/1
  SpdSet_dem2/1 -> Mux1/5
  Mux1/1 -> mot_lr/1
  TrqLim_dem2/1 -> Mux1/6
  HeartBeat1/1(life) -> Mux1/8, Memory1/1
  Memory1/1 -> HeartBeat1/1(life_pre)
  SpdLim_dem2/1 -> Mux1/7
  mot_drive3/1 -> Mux3/3
  mot_mode3/1 -> Mux3/2
  [trq_dem_rr1] -> Saturation3/1
  mot_enable3/1 -> Mux3/1
  SpdSet_dem3/1 -> Mux3/5
  Mux3/1 -> mot_rr/1
  TrqLim_dem3/1 -> Mux3/6
  SpdLim_dem3/1 -> Mux3/7
  bra_pre_l/1 -> Add9/2
  Add9/1 -> Saturation4/1
  1-D Lookup Table/1 -> Add9/1
  Constant/1 -> Product/1
  Product/1 -> Gain8/1
  Gain8/1 -> Gain11/1, Gain10/1
  Gain9/1 -> Product/2
  Gain10/1 -> 1-D Lookup Table/1
  Gain11/1 -> 1-D Lookup Table2/1
  1-D Lookup Table2/1 -> Add10/1
  bra_pre_r/1 -> Add10/2
  Add10/1 -> Saturation5/1
  brake_dem/1 -> Gain9/1
  Gain3/1 -> Difference/1
  Discrete-Time Integrator/1 -> Add2/2
  Difference/1 -> Add2/3
  Discrete-Time Integrator1/1 -> Add5/2
  Difference1/1 -> Add5/3
  Saturation/1 -> Mux/4
  Saturation1/1 -> Mux1/4
  Saturation2/1 -> Mux2/4
  Saturation3/1 -> Mux3/4
  Saturation4/1 -> bra_pre_l1/1
  Saturation5/1 -> bra_pre_r1/1
  Gain/1 -> Add6/1, Add3/1
  Gain12/1 -> Add6/2, Add4/1

== system DDCU_wxt_v02_forA_OpenLoop/MainControl/mode_control/forward/forward/Drive/驱动防滑控制TCS/转向TCS/右转/前轮滑转 ==
  trq_dem_lf : Inport
  trq_dem_lr : Inport  Port=2
  trq_dem_rf : Inport  Port=3
  trq_dem_rr : Inport  Port=4
  bra_pre_l : Inport  Port=5
  bra_pre_r : Inport  Port=6
  brake_dem : Inport  Port=7
  s_act_lf : Inport  Port=8
  s_opt_zhuan : Inport  Port=9
  Action Port : ActionPort  ActionType=case
  1-D Lookup Table : Lookup_n-D  NumberOfTableDimensions=1  BreakpointsForDimension1=brakeTrq_dem_data  Table=brakepre_dem_data  InternalRulePriority=Speed  RndMeth=Simplest  InputSameDT=on
  1-D Lookup Table2 : Lookup_n-D  NumberOfTableDimensions=1  BreakpointsForDimension1=brakeTrq_dem_data  Table=brakepre_dem_data  InternalRulePriority=Speed  RndMeth=Simplest  InputSameDT=on
  Add2 : Sum  Inputs=+++
  Add{3..6} (4 alike) : Sum
  Constant : Constant  Value=bratrq_max
  Difference : simulink/Discrete/Difference  ICPrevInput=0.0  InputProcessing=Inherited  OutMin=[]  OutMax=[]  OutDataType=fixdt(1, 16)  OutScaling=2^-10  DoSatur=off
  Discrete-Time Integrator : DiscreteIntegrator  SampleTime=-1  ICPrevOutput=DiscIntNeverNeededParam  ICPrevScaledInput=DiscIntNeverNeededParam
  Gain : Gain  Gain=1/tras_ratio
  Gain1 : Gain  Gain=kp2
  Gain2 : Gain  Gain=ki2
  Gain3 : Gain  Gain=kd2
  Gain4 : Gain  Gain=-1
  Gain5 : Gain  Gain=1/2
  Gain6 : Gain  Gain=1/100
  Gain7 : Gain  Gain=1/2
  Gain8 : Gain  Gain=1/2
  HeartBeat : MATLAB Function  TreatAsAtomicUnit=on
  HeartBeat1 : MATLAB Function  TreatAsAtomicUnit=on
  Memory : Memory  InheritSampleTime=on
  Memory1 : Memory  InheritSampleTime=on
  Mux : Mux  Inputs=8
  Mux1 : Mux  Inputs=8
  Mux2 : Mux  Inputs=7
  Mux3 : Mux  Inputs=7
  Product : Product
  Saturation{,1..3} (4 alike) : Saturate  UpperLimit=trqmax  LowerLimit=-trqmax
  Saturation4 : Saturate  UpperLimit=premax  LowerLimit=0
  Saturation5 : Saturate  UpperLimit=premax  LowerLimit=0
  SpdLim_dem{,1..3} (4 alike) : Constant  Value=spdmax
  SpdSet_dem{,1..3} (4 alike) : Constant
  Sum : Sum  Inputs=|+-
  TrqLim_dem{,1..3} (4 alike) : Constant
  mot_drive : Constant
  mot_drive1 : Constant  Value=2
  mot_drive2 : Constant
  mot_drive3 : Constant  Value=2
  mot_enable{,1..3} (4 alike) : Constant  Value=2
  mot_mode{,1..3} (4 alike) : Constant
  mot_lf : Outport
  mot_lr : Outport  Port=2
  mot_rf : Outport  Port=3
  mot_rr : Outport  Port=4
  bra_pre_l1 : Outport  Port=5
  bra_pre_r1 : Outport  Port=6
  wires:
  Add4/1 -> [trq_dem_lr1]
  trq_dem_lr/1 -> Add4/2
  Gain4/1 -> Add4/1
  Add3/1 -> [trq_dem_lf1]
  trq_dem_lf/1 -> Add3/2
  Add2/1 -> Gain/1
  s_act_lf/1 -> Sum/2
  Gain3/1 -> Difference/1
  Gain2/1 -> Discrete-Time Integrator/1
  Gain1/1 -> Add2/1
  Sum/1 -> Gain1/1, Gain3/1, Gain2/1
  s_opt_zhuan/1 -> Sum/1
  mot_drive/1 -> Mux/3
  mot_mode/1 -> Mux/2
  [trq_dem_lf1] -> Saturation/1
  mot_enable/1 -> Mux/1
  SpdSet_dem/1 -> Mux/5
  Mux/1 -> mot_lf/1
  TrqLim_dem/1 -> Mux/6
  HeartBeat/1(life) -> Mux/8, Memory/1
  Memory/1 -> HeartBeat/1(life_pre)
  SpdLim_dem/1 -> Mux/7
  mot_drive1/1 -> Mux2/3
  mot_mode2/1 -> Mux2/2
  trq_dem_rf/1 -> Saturation2/1
  mot_enable2/1 -> Mux2/1
  SpdSet_dem1/1 -> Mux2/5
  Mux2/1 -> mot_rf/1
  TrqLim_dem1/1 -> Mux2/6
  SpdLim_dem1/1 -> Mux2/7
  mot_drive2/1 -> Mux1/3
  mot_mode1/1 -> Mux1/2
  [trq_dem_lr1] -> Saturation1/1
  mot_enable1/1 -> Mux1/1
  SpdSet_dem2/1 -> Mux1/5
  Mux1/1 -> mot_lr/1
  TrqLim_dem2/1 -> Mux1/6
  HeartBeat1/1(life) -> Mux1/8, Memory1/1
  Memory1/1 -> HeartBeat1/1(life_pre)
  SpdLim_dem2/1 -> Mux1/7
  mot_drive3/1 -> Mux3/3
  mot_mode3/1 -> Mux3/2
  trq_dem_rr/1 -> Saturation3/1
  mot_enable3/1 -> Mux3/1
  SpdSet_dem3/1 -> Mux3/5
  Mux3/1 -> mot_rr/1
  TrqLim_dem3/1 -> Mux3/6
  SpdLim_dem3/1 -> Mux3/7
  bra_pre_l/1 -> Add5/2
  Add5/1 -> Saturation4/1
  1-D Lookup Table/1 -> Add5/1
  Constant/1 -> Product/1
  Product/1 -> Gain5/1
  Gain5/1 -> Gain8/1, Gain7/1
  Gain6/1 -> Product/2
  Gain7/1 -> 1-D Lookup Table/1
  Gain8/1 -> 1-D Lookup Table2/1
  1-D Lookup Table2/1 -> Add6/1
  bra_pre_r/1 -> Add6/2
  Add6/1 -> Saturation5/1
  brake_dem/1 -> Gain6/1
  Discrete-Time Integrator/1 -> Add2/2
  Difference/1 -> Add2/3
  Saturation/1 -> Mux/4
  Saturation1/1 -> Mux1/4
  Saturation2/1 -> Mux2/4
  Saturation3/1 -> Mux3/4
  Saturation4/1 -> bra_pre_l1/1
  Saturation5/1 -> bra_pre_r1/1
  Gain/1 -> Add3/1, Gain4/1

== system DDCU_wxt_v02_forA_OpenLoop/MainControl/mode_control/forward/forward/Drive/驱动防滑控制TCS/转向TCS/右转/后轮滑转 ==
  trq_dem_lf : Inport
  trq_dem_lr : Inport  Port=2
  trq_dem_rf : Inport  Port=3
  trq_dem_rr : Inport  Port=4
  bra_pre_l : Inport  Port=5
  bra_pre_r : Inport  Port=6
  brake_dem : Inport  Port=7
  s_act_lr : Inport  Port=8
  s_opt_zhuan : Inport  Port=9
  Action Port : ActionPort  ActionType=case
  1-D Lookup Table : Lookup_n-D  NumberOfTableDimensions=1  BreakpointsForDimension1=brakeTrq_dem_data  Table=brakepre_dem_data  InternalRulePriority=Speed  RndMeth=Simplest  InputSameDT=on
  1-D Lookup Table2 : Lookup_n-D  NumberOfTableDimensions=1  BreakpointsForDimension1=brakeTrq_dem_data  Table=brakepre_dem_data  InternalRulePriority=Speed  RndMeth=Simplest  InputSameDT=on
  Add2 : Sum  Inputs=+++
  Add{3..6} (4 alike) : Sum
  Constant : Constant  Value=bratrq_max
  Difference : simulink/Discrete/Difference  ICPrevInput=0.0  InputProcessing=Inherited  OutMin=[]  OutMax=[]  OutDataType=fixdt(1, 16)  OutScaling=2^-10  DoSatur=off
  Discrete-Time Integrator : DiscreteIntegrator  SampleTime=-1  ICPrevOutput=DiscIntNeverNeededParam  ICPrevScaledInput=DiscIntNeverNeededParam
  Gain : Gain  Gain=1/tras_ratio
  Gain1 : Gain  Gain=kp2
  Gain2 : Gain  Gain=ki2
  Gain3 : Gain  Gain=kd2
  Gain4 : Gain  Gain=-1
  Gain5 : Gain  Gain=1/2
  Gain6 : Gain  Gain=1/100
  Gain7 : Gain  Gain=1/2
  Gain8 : Gain  Gain=1/2
  HeartBeat : MATLAB Function  TreatAsAtomicUnit=on
  HeartBeat1 : MATLAB Function  TreatAsAtomicUnit=on
  Memory : Memory  InheritSampleTime=on
  Memory1 : Memory  InheritSampleTime=on
  Mux : Mux  Inputs=8
  Mux1 : Mux  Inputs=8
  Mux2 : Mux  Inputs=7
  Mux3 : Mux  Inputs=7
  Product : Product
  Saturation{,1..3} (4 alike) : Saturate  UpperLimit=trqmax  LowerLimit=-trqmax
  Saturation4 : Saturate  UpperLimit=premax  LowerLimit=0
  Saturation5 : Saturate  UpperLimit=premax  LowerLimit=0
  SpdLim_dem{,1..3} (4 alike) : Constant  Value=spdmax
  SpdSet_dem{,1..3} (4 alike) : Constant
  Sum : Sum  Inputs=|+-
  TrqLim_dem{,1..3} (4 alike) : Constant
  mot_drive : Constant
  mot_drive1 : Constant  Value=2
  mot_drive2 : Constant
  mot_drive3 : Constant  Value=2
  mot_enable{,1..3} (4 alike) : Constant  Value=2
  mot_mode{,1..3} (4 alike) : Constant
  mot_lf : Outport
  mot_lr : Outport  Port=2
  mot_rf : Outport  Port=3
  mot_rr : Outport  Port=4
  bra_pre_l1 : Outport  Port=5
  bra_pre_r1 : Outport  Port=6
  wires:
  SpdLim_dem3/1 -> Mux3/7
  TrqLim_dem3/1 -> Mux3/6
  Mux3/1 -> mot_rr/1
  SpdSet_dem3/1 -> Mux3/5
  mot_enable3/1 -> Mux3/1
  trq_dem_rr/1 -> Saturation3/1
  mot_mode3/1 -> Mux3/2
  mot_drive3/1 -> Mux3/3
  SpdLim_dem2/1 -> Mux1/7
  Memory1/1 -> HeartBeat1/1(life_pre)
  HeartBeat1/1(life) -> Memory1/1, Mux1/8
  TrqLim_dem2/1 -> Mux1/6
  Mux1/1 -> mot_lr/1
  SpdSet_dem2/1 -> Mux1/5
  mot_enable1/1 -> Mux1/1
  [trq_dem_lr1] -> Saturation1/1
  mot_mode1/1 -> Mux1/2
  mot_drive2/1 -> Mux1/3
  SpdLim_dem1/1 -> Mux2/7
  TrqLim_dem1/1 -> Mux2/6
  Mux2/1 -> mot_rf/1
  SpdSet_dem1/1 -> Mux2/5
  mot_enable2/1 -> Mux2/1
  trq_dem_rf/1 -> Saturation2/1
  mot_mode2/1 -> Mux2/2
  mot_drive1/1 -> Mux2/3
  SpdLim_dem/1 -> Mux/7
  Memory/1 -> HeartBeat/1(life_pre)
  HeartBeat/1(life) -> Memory/1, Mux/8
  TrqLim_dem/1 -> Mux/6
  Mux/1 -> mot_lf/1
  SpdSet_dem/1 -> Mux/5
  mot_enable/1 -> Mux/1
  [trq_dem_lf1] -> Saturation/1
  mot_mode/1 -> Mux/2
  mot_drive/1 -> Mux/3
  s_opt_zhuan/1 -> Sum/1
  Sum/1 -> Gain2/1, Gain3/1, Gain1/1
  Gain1/1 -> Add2/1
  Gain2/1 -> Discrete-Time Integrator/1
  Gain3/1 -> Difference/1
  s_act_lr/1 -> Sum/2
  Add2/1 -> Gain/1
  trq_dem_lr/1 -> Add3/2
  Add3/1 -> [trq_dem_lr1]
  Gain4/1 -> Add4/1
  trq_dem_lf/1 -> Add4/2
  Add4/1 -> [trq_dem_lf1]
  bra_pre_l/1 -> Add5/2
  Add5/1 -> Saturation4/1
  1-D Lookup Table/1 -> Add5/1
  Constant/1 -> Product/1
  Product/1 -> Gain5/1
  Gain5/1 -> Gain8/1, Gain7/1
  Gain6/1 -> Product/2
  Gain7/1 -> 1-D Lookup Table/1
  Gain8/1 -> 1-D Lookup Table2/1
  1-D Lookup Table2/1 -> Add6/1
  bra_pre_r/1 -> Add6/2
  Add6/1 -> Saturation5/1
  brake_dem/1 -> Gain6/1
  Discrete-Time Integrator/1 -> Add2/2
  Difference/1 -> Add2/3
  Saturation/1 -> Mux/4
  Saturation1/1 -> Mux1/4
  Saturation2/1 -> Mux2/4
  Saturation3/1 -> Mux3/4
  Saturation4/1 -> bra_pre_l1/1
  Saturation5/1 -> bra_pre_r1/1
  Gain/1 -> Gain4/1, Add3/1

== system DDCU_wxt_v02_forA_OpenLoop/MainControl/mode_control/forward/forward/Drive/驱动防滑控制TCS/转向TCS/右转/无滑转 ==
  trq_dem_lf : Inport
  trq_dem_lr : Inport  Port=2
  trq_dem_rf : Inport  Port=3
  trq_dem_rr : Inport  Port=4
  bra_pre_l : Inport  Port=5
  bra_pre_r : Inport  Port=6
  brake_dem : Inport  Port=7
  Action Port : ActionPort  ActionType=case
  1-D Lookup Table : Lookup_n-D  NumberOfTableDimensions=1  BreakpointsForDimension1=brakeTrq_dem_data  Table=brakepre_dem_data  InternalRulePriority=Speed  RndMeth=Simplest  InputSameDT=on
  1-D Lookup Table2 : Lookup_n-D  NumberOfTableDimensions=1  BreakpointsForDimension1=brakeTrq_dem_data  Table=brakepre_dem_data  InternalRulePriority=Speed  RndMeth=Simplest  InputSameDT=on
  Add2 : Sum
  Add3 : Sum
  Constant : Constant  Value=bratrq_max
  Gain1 : Gain  Gain=1/2
  Gain2 : Gain  Gain=1/100
  Gain3 : Gain  Gain=1/2
  Gain4 : Gain  Gain=1/2
  HeartBeat : MATLAB Function  TreatAsAtomicUnit=on
  HeartBeat1 : MATLAB Function  TreatAsAtomicUnit=on
  Memory : Memory  InheritSampleTime=on
  Memory1 : Memory  InheritSampleTime=on
  Mux : Mux  Inputs=8
  Mux1 : Mux  Inputs=8
  Mux2 : Mux  Inputs=7
  Mux3 : Mux  Inputs=7
  Product : Product
  Saturation{,1..3} (4 alike) : Saturate  UpperLimit=trqmax  LowerLimit=-trqmax
  Saturation4 : Saturate  UpperLimit=premax  LowerLimit=0
  Saturation5 : Saturate  UpperLimit=premax  LowerLimit=0
  SpdLim_dem{,1..3} (4 alike) : Constant  Value=spdmax
  SpdSet_dem{,1..3} (4 alike) : Constant
  TrqLim_dem{,1..3} (4 alike) : Constant
  mot_drive : Constant
  mot_drive1 : Constant  Value=2
  mot_drive2 : Constant
  mot_drive3 : Constant  Value=2
  mot_enable{,1..3} (4 alike) : Constant  Value=2
  mot_mode{,1..3} (4 alike) : Constant
  mot_lf : Outport
  mot_lr : Outport  Port=2
  mot_rf : Outport  Port=3
  mot_rr : Outport  Port=4
  bra_pre_l1 : Outport  Port=5
  bra_pre_r1 : Outport  Port=6
  wires:
  SpdLim_dem3/1 -> Mux3/7
  TrqLim_dem3/1 -> Mux3/6
  Mux3/1 -> mot_rr/1
  SpdSet_dem3/1 -> Mux3/5
  mot_enable3/1 -> Mux3/1
  trq_dem_rr/1 -> Saturation3/1
  mot_mode3/1 -> Mux3/2
  mot_drive3/1 -> Mux3/3
  SpdLim_dem2/1 -> Mux1/7
  Memory1/1 -> HeartBeat1/1(life_pre)
  HeartBeat1/1(life) -> Memory1/1, Mux1/8
  TrqLim_dem2/1 -> Mux1/6
  Mux1/1 -> mot_lr/1
  SpdSet_dem2/1 -> Mux1/5
  mot_enable1/1 -> Mux1/1
  trq_dem_lr/1 -> Saturation1/1
  mot_mode1/1 -> Mux1/2
  mot_drive2/1 -> Mux1/3
  SpdLim_dem1/1 -> Mux2/7
  TrqLim_dem1/1 -> Mux2/6
  Mux2/1 -> mot_rf/1
  SpdSet_dem1/1 -> Mux2/5
  mot_enable2/1 -> Mux2/1
  trq_dem_rf/1 -> Saturation2/1
  mot_mode2/1 -> Mux2/2
  mot_drive1/1 -> Mux2/3
  SpdLim_dem/1 -> Mux/7
  Memory/1 -> HeartBeat/1(life_pre)
  HeartBeat/1(life) -> Memory/1, Mux/8
  TrqLim_dem/1 -> Mux/6
  Mux/1 -> mot_lf/1
  SpdSet_dem/1 -> Mux/5
  mot_enable/1 -> Mux/1
  trq_dem_lf/1 -> Saturation/1
  mot_mode/1 -> Mux/2
  mot_drive/1 -> Mux/3
  bra_pre_l/1 -> Add2/2
  Add2/1 -> Saturation4/1
  1-D Lookup Table/1 -> Add2/1
  Constant/1 -> Product/1
  Product/1 -> Gain1/1
  Gain1/1 -> Gain4/1, Gain3/1
  Gain2/1 -> Product/2
  Gain3/1 -> 1-D Lookup Table/1
  Gain4/1 -> 1-D Lookup Table2/1
  1-D Lookup Table2/1 -> Add3/1
  bra_pre_r/1 -> Add3/2
  Add3/1 -> Saturation5/1
  brake_dem/1 -> Gain2/1
  Saturation/1 -> Mux/4
  Saturation1/1 -> Mux1/4
  Saturation2/1 -> Mux2/4
  Saturation3/1 -> Mux3/4
  Saturation4/1 -> bra_pre_l1/1
  Saturation5/1 -> bra_pre_r1/1

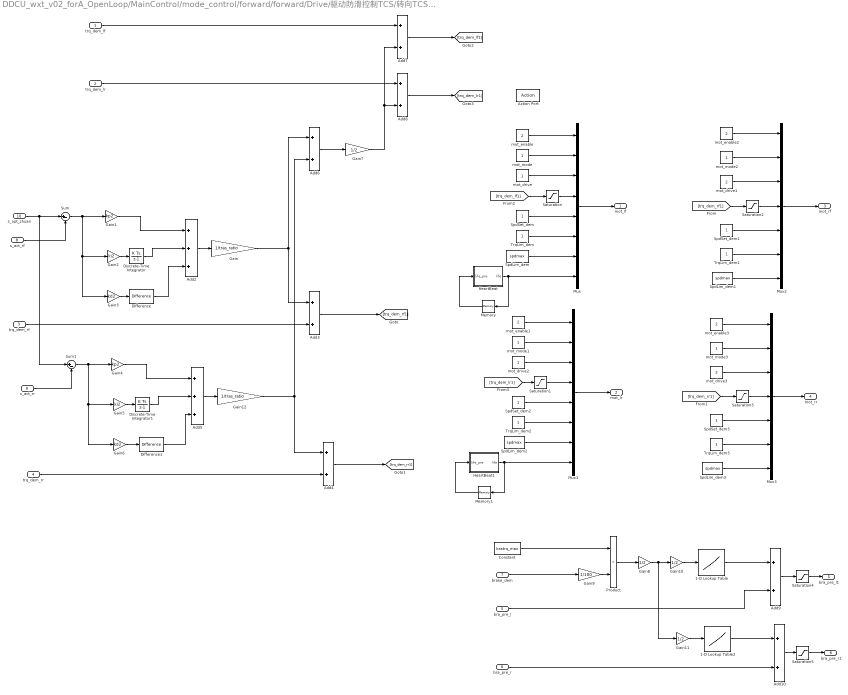
== system DDCU_wxt_v02_forA_OpenLoop/MainControl/mode_control/forward/forward/Drive/驱动防滑控制TCS/转向TCS/左转/前后轮均滑转 ==
  trq_dem_lf : Inport
  trq_dem_lr : Inport  Port=2
  trq_dem_rf : Inport  Port=3
  trq_dem_rr : Inport  Port=4
  bra_pre_l : Inport  Port=5
  bra_pre_r : Inport  Port=6
  brake_dem : Inport  Port=7
  s_act_rf : Inport  Port=8
  s_act_rr : Inport  Port=9
  s_opt_zhuan : Inport  Port=10
  Action Port : ActionPort  ActionType=case
  1-D Lookup Table : Lookup_n-D  NumberOfTableDimensions=1  BreakpointsForDimension1=brakeTrq_dem_data  Table=brakepre_dem_data  InternalRulePriority=Speed  RndMeth=Simplest  InputSameDT=on
  1-D Lookup Table2 : Lookup_n-D  NumberOfTableDimensions=1  BreakpointsForDimension1=brakeTrq_dem_data  Table=brakepre_dem_data  InternalRulePriority=Speed  RndMeth=Simplest  InputSameDT=on
  Add{3..4,6..10} (7 alike) : Sum
  Add2 : Sum  Inputs=+++
  Add5 : Sum  Inputs=+++
  Constant : Constant  Value=bratrq_max
  Difference : simulink/Discrete/Difference  ICPrevInput=0.0  InputProcessing=Inherited  OutMin=[]  OutMax=[]  OutDataType=fixdt(1, 16)  OutScaling=2^-10  DoSatur=off
  Difference1 : simulink/Discrete/Difference  ICPrevInput=0.0  InputProcessing=Inherited  OutMin=[]  OutMax=[]  OutDataType=fixdt(1, 16)  OutScaling=2^-10  DoSatur=off
  Discrete-Time Integrator : DiscreteIntegrator  SampleTime=-1  ICPrevOutput=DiscIntNeverNeededParam  ICPrevScaledInput=DiscIntNeverNeededParam
  Discrete-Time Integrator1 : DiscreteIntegrator  SampleTime=-1  ICPrevOutput=DiscIntNeverNeededParam  ICPrevScaledInput=DiscIntNeverNeededParam
  Gain : Gain  Gain=1/tras_ratio
  Gain1 : Gain  Gain=kp2
  Gain{7..8,10..11} (4 alike) : Gain  Gain=1/2
  Gain12 : Gain  Gain=1/tras_ratio
  Gain2 : Gain  Gain=ki2
  Gain3 : Gain  Gain=kd2
  Gain4 : Gain  Gain=kp2
  Gain5 : Gain  Gain=ki2
  Gain6 : Gain  Gain=kd2
  Gain9 : Gain  Gain=1/100
  HeartBeat : MATLAB Function  TreatAsAtomicUnit=on
  HeartBeat1 : MATLAB Function  TreatAsAtomicUnit=on
  Memory : Memory  InheritSampleTime=on
  Memory1 : Memory  InheritSampleTime=on
  Mux : Mux  Inputs=8
  Mux1 : Mux  Inputs=8
  Mux2 : Mux  Inputs=7
  Mux3 : Mux  Inputs=7
  Product : Product
  Saturation{,1..3} (4 alike) : Saturate  UpperLimit=trqmax  LowerLimit=-trqmax
  Saturation4 : Saturate  UpperLimit=premax  LowerLimit=0
  Saturation5 : Saturate  UpperLimit=premax  LowerLimit=0
  SpdLim_dem{,1..3} (4 alike) : Constant  Value=spdmax
  SpdSet_dem{,1..3} (4 alike) : Constant
  Sum : Sum  Inputs=|+-
  Sum1 : Sum  Inputs=|+-
  TrqLim_dem{,1..3} (4 alike) : Constant
  mot_drive : Constant
  mot_drive1 : Constant  Value=2
  mot_drive2 : Constant
  mot_drive3 : Constant  Value=2
  mot_enable{,1..3} (4 alike) : Constant  Value=2
  mot_mode{,1..3} (4 alike) : Constant
  mot_lf : Outport
  mot_lr : Outport  Port=2
  mot_rf : Outport  Port=3
  mot_rr : Outport  Port=4
  bra_pre_l1 : Outport  Port=5
  bra_pre_r1 : Outport  Port=6
  wires:
  SpdLim_dem3/1 -> Mux3/7
  TrqLim_dem3/1 -> Mux3/6
  Mux3/1 -> mot_rr/1
  SpdSet_dem3/1 -> Mux3/5
  mot_enable3/1 -> Mux3/1
  [trq_dem_rr1] -> Saturation3/1
  mot_mode3/1 -> Mux3/2
  mot_drive3/1 -> Mux3/3
  SpdLim_dem2/1 -> Mux1/7
  Memory1/1 -> HeartBeat1/1(life_pre)
  HeartBeat1/1(life) -> Memory1/1, Mux1/8
  TrqLim_dem2/1 -> Mux1/6
  Mux1/1 -> mot_lr/1
  SpdSet_dem2/1 -> Mux1/5
  mot_enable1/1 -> Mux1/1
  [trq_dem_lr1] -> Saturation1/1
  mot_mode1/1 -> Mux1/2
  mot_drive2/1 -> Mux1/3
  SpdLim_dem1/1 -> Mux2/7
  TrqLim_dem1/1 -> Mux2/6
  Mux2/1 -> mot_rf/1
  SpdSet_dem1/1 -> Mux2/5
  mot_enable2/1 -> Mux2/1
  [trq_dem_rf1] -> Saturation2/1
  mot_mode2/1 -> Mux2/2
  mot_drive1/1 -> Mux2/3
  SpdLim_dem/1 -> Mux/7
  Memory/1 -> HeartBeat/1(life_pre)
  HeartBeat/1(life) -> Memory/1, Mux/8
  TrqLim_dem/1 -> Mux/6
  Mux/1 -> mot_lf/1
  SpdSet_dem/1 -> Mux/5
  mot_enable/1 -> Mux/1
  [trq_dem_lf1] -> Saturation/1
  mot_mode/1 -> Mux/2
  mot_drive/1 -> Mux/3
  s_opt_zhuan/1 -> Sum1/1, Sum/1
  Sum/1 -> Gain2/1, Gain3/1, Gain1/1
  Gain1/1 -> Add2/1
  Gain2/1 -> Discrete-Time Integrator/1
  Gain3/1 -> Difference/1
  s_act_rf/1 -> Sum/2
  Add2/1 -> Gain/1
  trq_dem_rf/1 -> Add3/2
  Add3/1 -> [trq_dem_rf1]
  Add4/1 -> [trq_dem_rr1]
  Sum1/1 -> Gain5/1, Gain6/1, Gain4/1
  Gain4/1 -> Add5/1
  Gain5/1 -> Discrete-Time Integrator1/1
  Gain6/1 -> Difference1/1
  s_act_rr/1 -> Sum1/2
  Add5/1 -> Gain12/1
  trq_dem_rr/1 -> Add4/2
  Add6/1 -> Gain7/1
  trq_dem_lf/1 -> Add7/1
  Gain7/1 -> Add8/2, Add7/2
  Add7/1 -> [trq_dem_lf1]
  trq_dem_lr/1 -> Add8/1
  Add8/1 -> [trq_dem_lr1]
  bra_pre_l/1 -> Add9/2
  Add9/1 -> Saturation4/1
  1-D Lookup Table/1 -> Add9/1
  Constant/1 -> Product/1
  Product/1 -> Gain8/1
  Gain8/1 -> Gain11/1, Gain10/1
  Gain9/1 -> Product/2
  Gain10/1 -> 1-D Lookup Table/1
  Gain11/1 -> 1-D Lookup Table2/1
  1-D Lookup Table2/1 -> Add10/1
  bra_pre_r/1 -> Add10/2
  Add10/1 -> Saturation5/1
  brake_dem/1 -> Gain9/1
  Discrete-Time Integrator/1 -> Add2/2
  Difference/1 -> Add2/3
  Discrete-Time Integrator1/1 -> Add5/2
  Difference1/1 -> Add5/3
  Saturation/1 -> Mux/4
  Saturation1/1 -> Mux1/4
  Saturation2/1 -> Mux2/4
  Saturation3/1 -> Mux3/4
  Saturation4/1 -> bra_pre_l1/1
  Saturation5/1 -> bra_pre_r1/1
  Gain/1 -> Add3/1, Add6/1
  Gain12/1 -> Add4/1, Add6/2

== matlab function DDCU_wxt_v02_forA_OpenLoop/MainControl/mode_control/emergency_stop/emergency_stop/HeartBeat1 ==
  data: life_pre input; life output
function life = fcn(life_pre)
%#codegen
life=life_pre+1;
if life>15
    life=0;
end
end

== matlab function DDCU_wxt_v02_forA_OpenLoop/MainControl/mode_control/backward/backward/Brake/MATLAB Function1 ==
  data: syi_act_lf input; flagyi_lf output; s_opt_yi input; s_opt_yi_add input; flagyi_lf_pre input
function flagyi_lf = fcn(syi_act_lf,s_opt_yi,s_opt_yi_add,flagyi_lf_pre)
%#codegen
if syi_act_lf>s_opt_yi+s_opt_yi_add
    flagyi_lf=1;
elseif syi_act_lf<s_opt_yi
    flagyi_lf = 0;
else
    flagyi_lf=flagyi_lf_pre;
end
end
